simulink model "c00016M_harness"  (R2018a)
settings: Solver=FixedStepAuto  StartTime=0.0  StopTime=300  FixedStep=0.1  RelTol=1e-3
undefined symbols (not defined in the file): A1, hmax, PriorityTank, R1, R2, sigbuilder_block
(part 4 of 24)

== system c00016M_harness/M092 ==
  note: VALUES
      | ---------------------------------
      | ControlType = 1 | 2 | 3
      | FillTank = 0 | 1
      | EmptyTank = 0 | 1
      | ManualReference between 0 and 1
      | Tempreature between 0 and 100
      | EmergencyButton = 0 | 1
      | LiquidLevel between 0 and 1 (hmax)
  note: Inputs For Tank2
  note: NAMES
      | --------------------------------------------
      | CT1 = ControlType Tank 1
      | F1 = Fill Tank 1
      | E1 = Empty Tank 1
      | MR1 = Manual Reference Tank1
      | T1 = Temperature Tank 1
      | EB1 = Emergency Button Tank 1
      | LL1 = Liquid Level 1
  note: Inputs For Tank3
  note: Inputs For Tank1
  CT2 : Inport
  T2 : Inport  Port=2
  EB2 : Inport  Port=3
  CT3 : Inport  Port=4
  F3 : Inport  Port=5
  E3 : Inport  Port=6
  T3 : Inport  Port=7
  EB3 : Inport  Port=8
  Tank2 : Subsystem
  Tank3 : Subsystem
  LL2 : Outport
  LL3 : Outport  Port=2
  wires:
  Tank2/1(LL2) -> LL2/1, Tank3/6(LL2)
  Tank3/1(LL3) -> LL3/1, Tank2/4(LL3)
  EB2/1 -> Tank2/3(EB2)
  CT2/1 -> Tank2/1(CT2)
  E3/1 -> Tank3/3(E3)
  T2/1 -> Tank2/2(T2)
  CT3/1 -> Tank3/1(CT3)
  F3/1 -> Tank3/2(F3)
  EB3/1 -> Tank3/5(EB3)
  T3/1 -> Tank3/4(T3)

== system c00016M_harness/M093 ==
  note: VALUES
      | ---------------------------------
      | ControlType = 1 | 2 | 3
      | FillTank = 0 | 1
      | EmptyTank = 0 | 1
      | ManualReference between 0 and 1
      | Tempreature between 0 and 100
      | EmergencyButton = 0 | 1
      | LiquidLevel between 0 and 1 (hmax)
  note: Inputs For Tank2
  note: NAMES
      | --------------------------------------------
      | CT1 = ControlType Tank 1
      | F1 = Fill Tank 1
      | E1 = Empty Tank 1
      | MR1 = Manual Reference Tank1
      | T1 = Temperature Tank 1
      | EB1 = Emergency Button Tank 1
      | LL1 = Liquid Level 1
  note: Inputs For Tank3
  note: Inputs For Tank1
  CT2 : Inport
  T2 : Inport  Port=2
  EB2 : Inport  Port=3
  CT3 : Inport  Port=4
  F3 : Inport  Port=5
  E3 : Inport  Port=6
  T3 : Inport  Port=7
  EB3 : Inport  Port=8
  Tank2 : Subsystem
  Tank3 : Subsystem
  LL2 : Outport
  LL3 : Outport  Port=2
  wires:
  Tank2/1(LL2) -> LL2/1, Tank3/6(LL2)
  Tank3/1(LL3) -> LL3/1, Tank2/4(LL3)
  EB2/1 -> Tank2/3(EB2)
  CT2/1 -> Tank2/1(CT2)
  E3/1 -> Tank3/3(E3)
  T2/1 -> Tank2/2(T2)
  CT3/1 -> Tank3/1(CT3)
  F3/1 -> Tank3/2(F3)
  EB3/1 -> Tank3/5(EB3)
  T3/1 -> Tank3/4(T3)

== system c00016M_harness/M094 ==
  note: VALUES
      | ---------------------------------
      | ControlType = 1 | 2 | 3
      | FillTank = 0 | 1
      | EmptyTank = 0 | 1
      | ManualReference between 0 and 1
      | Tempreature between 0 and 100
      | EmergencyButton = 0 | 1
      | LiquidLevel between 0 and 1 (hmax)
  note: Inputs For Tank2
  note: NAMES
      | --------------------------------------------
      | CT1 = ControlType Tank 1
      | F1 = Fill Tank 1
      | E1 = Empty Tank 1
      | MR1 = Manual Reference Tank1
      | T1 = Temperature Tank 1
      | EB1 = Emergency Button Tank 1
      | LL1 = Liquid Level 1
  note: Inputs For Tank3
  note: Inputs For Tank1
  CT2 : Inport
  T2 : Inport  Port=2
  EB2 : Inport  Port=3
  CT3 : Inport  Port=4
  F3 : Inport  Port=5
  E3 : Inport  Port=6
  T3 : Inport  Port=7
  EB3 : Inport  Port=8
  Tank2 : Subsystem
  Tank3 : Subsystem
  LL2 : Outport
  LL3 : Outport  Port=2
  wires:
  Tank2/1(LL2) -> LL2/1, Tank3/6(LL2)
  Tank3/1(LL3) -> LL3/1, Tank2/4(LL3)
  EB2/1 -> Tank2/3(EB2)
  CT2/1 -> Tank2/1(CT2)
  E3/1 -> Tank3/3(E3)
  T2/1 -> Tank2/2(T2)
  CT3/1 -> Tank3/1(CT3)
  F3/1 -> Tank3/2(F3)
  EB3/1 -> Tank3/5(EB3)
  T3/1 -> Tank3/4(T3)

== system c00016M_harness/M095 ==
  note: VALUES
      | ---------------------------------
      | ControlType = 1 | 2 | 3
      | FillTank = 0 | 1
      | EmptyTank = 0 | 1
      | ManualReference between 0 and 1
      | Tempreature between 0 and 100
      | EmergencyButton = 0 | 1
      | LiquidLevel between 0 and 1 (hmax)
  note: Inputs For Tank2
  note: NAMES
      | --------------------------------------------
      | CT1 = ControlType Tank 1
      | F1 = Fill Tank 1
      | E1 = Empty Tank 1
      | MR1 = Manual Reference Tank1
      | T1 = Temperature Tank 1
      | EB1 = Emergency Button Tank 1
      | LL1 = Liquid Level 1
  note: Inputs For Tank3
  note: Inputs For Tank1
  CT2 : Inport
  T2 : Inport  Port=2
  EB2 : Inport  Port=3
  CT3 : Inport  Port=4
  F3 : Inport  Port=5
  E3 : Inport  Port=6
  T3 : Inport  Port=7
  EB3 : Inport  Port=8
  Tank2 : Subsystem
  Tank3 : Subsystem
  LL2 : Outport
  LL3 : Outport  Port=2
  wires:
  Tank2/1(LL2) -> LL2/1, Tank3/6(LL2)
  Tank3/1(LL3) -> LL3/1, Tank2/4(LL3)
  EB2/1 -> Tank2/3(EB2)
  CT2/1 -> Tank2/1(CT2)
  E3/1 -> Tank3/3(E3)
  T2/1 -> Tank2/2(T2)
  CT3/1 -> Tank3/1(CT3)
  F3/1 -> Tank3/2(F3)
  EB3/1 -> Tank3/5(EB3)
  T3/1 -> Tank3/4(T3)

== system c00016M_harness/M096 ==
  note: VALUES
      | ---------------------------------
      | ControlType = 1 | 2 | 3
      | FillTank = 0 | 1
      | EmptyTank = 0 | 1
      | ManualReference between 0 and 1
      | Tempreature between 0 and 100
      | EmergencyButton = 0 | 1
      | LiquidLevel between 0 and 1 (hmax)
  note: Inputs For Tank2
  note: NAMES
      | --------------------------------------------
      | CT1 = ControlType Tank 1
      | F1 = Fill Tank 1
      | E1 = Empty Tank 1
      | MR1 = Manual Reference Tank1
      | T1 = Temperature Tank 1
      | EB1 = Emergency Button Tank 1
      | LL1 = Liquid Level 1
  note: Inputs For Tank3
  note: Inputs For Tank1
  CT2 : Inport
  T2 : Inport  Port=2
  EB2 : Inport  Port=3
  CT3 : Inport  Port=4
  F3 : Inport  Port=5
  E3 : Inport  Port=6
  T3 : Inport  Port=7
  EB3 : Inport  Port=8
  Tank2 : Subsystem
  Tank3 : Subsystem
  LL2 : Outport
  LL3 : Outport  Port=2
  wires:
  Tank2/1(LL2) -> LL2/1, Tank3/6(LL2)
  Tank3/1(LL3) -> LL3/1, Tank2/4(LL3)
  EB2/1 -> Tank2/3(EB2)
  CT2/1 -> Tank2/1(CT2)
  E3/1 -> Tank3/3(E3)
  T2/1 -> Tank2/2(T2)
  CT3/1 -> Tank3/1(CT3)
  F3/1 -> Tank3/2(F3)
  EB3/1 -> Tank3/5(EB3)
  T3/1 -> Tank3/4(T3)

== system c00016M_harness/M097 ==
  note: VALUES
      | ---------------------------------
      | ControlType = 1 | 2 | 3
      | FillTank = 0 | 1
      | EmptyTank = 0 | 1
      | ManualReference between 0 and 1
      | Tempreature between 0 and 100
      | EmergencyButton = 0 | 1
      | LiquidLevel between 0 and 1 (hmax)
  note: Inputs For Tank2
  note: NAMES
      | --------------------------------------------
      | CT1 = ControlType Tank 1
      | F1 = Fill Tank 1
      | E1 = Empty Tank 1
      | MR1 = Manual Reference Tank1
      | T1 = Temperature Tank 1
      | EB1 = Emergency Button Tank 1
      | LL1 = Liquid Level 1
  note: Inputs For Tank3
  note: Inputs For Tank1
  CT2 : Inport
  T2 : Inport  Port=2
  EB2 : Inport  Port=3
  CT3 : Inport  Port=4
  F3 : Inport  Port=5
  E3 : Inport  Port=6
  T3 : Inport  Port=7
  EB3 : Inport  Port=8
  Tank2 : Subsystem
  Tank3 : Subsystem
  LL2 : Outport
  LL3 : Outport  Port=2
  wires:
  Tank2/1(LL2) -> LL2/1, Tank3/6(LL2)
  Tank3/1(LL3) -> LL3/1, Tank2/4(LL3)
  EB2/1 -> Tank2/3(EB2)
  CT2/1 -> Tank2/1(CT2)
  E3/1 -> Tank3/3(E3)
  T2/1 -> Tank2/2(T2)
  CT3/1 -> Tank3/1(CT3)
  F3/1 -> Tank3/2(F3)
  EB3/1 -> Tank3/5(EB3)
  T3/1 -> Tank3/4(T3)

== system c00016M_harness/M098 ==
  note: VALUES
      | ---------------------------------
      | ControlType = 1 | 2 | 3
      | FillTank = 0 | 1
      | EmptyTank = 0 | 1
      | ManualReference between 0 and 1
      | Tempreature between 0 and 100
      | EmergencyButton = 0 | 1
      | LiquidLevel between 0 and 1 (hmax)
  note: Inputs For Tank2
  note: NAMES
      | --------------------------------------------
      | CT1 = ControlType Tank 1
      | F1 = Fill Tank 1
      | E1 = Empty Tank 1
      | MR1 = Manual Reference Tank1
      | T1 = Temperature Tank 1
      | EB1 = Emergency Button Tank 1
      | LL1 = Liquid Level 1
  note: Inputs For Tank3
  note: Inputs For Tank1
  CT2 : Inport
  T2 : Inport  Port=2
  EB2 : Inport  Port=3
  CT3 : Inport  Port=4
  F3 : Inport  Port=5
  E3 : Inport  Port=6
  T3 : Inport  Port=7
  EB3 : Inport  Port=8
  Tank2 : Subsystem
  Tank3 : Subsystem
  LL2 : Outport
  LL3 : Outport  Port=2
  wires:
  Tank2/1(LL2) -> LL2/1, Tank3/6(LL2)
  Tank3/1(LL3) -> LL3/1, Tank2/4(LL3)
  EB2/1 -> Tank2/3(EB2)
  CT2/1 -> Tank2/1(CT2)
  E3/1 -> Tank3/3(E3)
  T2/1 -> Tank2/2(T2)
  CT3/1 -> Tank3/1(CT3)
  F3/1 -> Tank3/2(F3)
  EB3/1 -> Tank3/5(EB3)
  T3/1 -> Tank3/4(T3)

== system c00016M_harness/M099 ==
  note: VALUES
      | ---------------------------------
      | ControlType = 1 | 2 | 3
      | FillTank = 0 | 1
      | EmptyTank = 0 | 1
      | ManualReference between 0 and 1
      | Tempreature between 0 and 100
      | EmergencyButton = 0 | 1
      | LiquidLevel between 0 and 1 (hmax)
  note: Inputs For Tank2
  note: NAMES
      | --------------------------------------------
      | CT1 = ControlType Tank 1
      | F1 = Fill Tank 1
      | E1 = Empty Tank 1
      | MR1 = Manual Reference Tank1
      | T1 = Temperature Tank 1
      | EB1 = Emergency Button Tank 1
      | LL1 = Liquid Level 1
  note: Inputs For Tank3
  note: Inputs For Tank1
  CT2 : Inport
  T2 : Inport  Port=2
  EB2 : Inport  Port=3
  CT3 : Inport  Port=4
  F3 : Inport  Port=5
  E3 : Inport  Port=6
  T3 : Inport  Port=7
  EB3 : Inport  Port=8
  Tank2 : Subsystem
  Tank3 : Subsystem
  LL2 : Outport
  LL3 : Outport  Port=2
  wires:
  Tank2/1(LL2) -> LL2/1, Tank3/6(LL2)
  Tank3/1(LL3) -> LL3/1, Tank2/4(LL3)
  EB2/1 -> Tank2/3(EB2)
  CT2/1 -> Tank2/1(CT2)
  E3/1 -> Tank3/3(E3)
  T2/1 -> Tank2/2(T2)
  CT3/1 -> Tank3/1(CT3)
  F3/1 -> Tank3/2(F3)
  EB3/1 -> Tank3/5(EB3)
  T3/1 -> Tank3/4(T3)

== system c00016M_harness/M100 ==
  note: VALUES
      | ---------------------------------
      | ControlType = 1 | 2 | 3
      | FillTank = 0 | 1
      | EmptyTank = 0 | 1
      | ManualReference between 0 and 1
      | Tempreature between 0 and 100
      | EmergencyButton = 0 | 1
      | LiquidLevel between 0 and 1 (hmax)
  note: Inputs For Tank2
  note: NAMES
      | --------------------------------------------
      | CT1 = ControlType Tank 1
      | F1 = Fill Tank 1
      | E1 = Empty Tank 1
      | MR1 = Manual Reference Tank1
      | T1 = Temperature Tank 1
      | EB1 = Emergency Button Tank 1
      | LL1 = Liquid Level 1
  note: Inputs For Tank3
  note: Inputs For Tank1
  CT2 : Inport
  T2 : Inport  Port=2
  EB2 : Inport  Port=3
  CT3 : Inport  Port=4
  F3 : Inport  Port=5
  E3 : Inport  Port=6
  T3 : Inport  Port=7
  EB3 : Inport  Port=8
  Tank2 : Subsystem
  Tank3 : Subsystem
  LL2 : Outport
  LL3 : Outport  Port=2
  wires:
  Tank2/1(LL2) -> LL2/1, Tank3/6(LL2)
  Tank3/1(LL3) -> LL3/1, Tank2/4(LL3)
  EB2/1 -> Tank2/3(EB2)
  CT2/1 -> Tank2/1(CT2)
  E3/1 -> Tank3/3(E3)
  T2/1 -> Tank2/2(T2)
  CT3/1 -> Tank3/1(CT3)
  F3/1 -> Tank3/2(F3)
  EB3/1 -> Tank3/5(EB3)
  T3/1 -> Tank3/4(T3)

== system c00016M_harness/M101 ==
  note: VALUES
      | ---------------------------------
      | ControlType = 1 | 2 | 3
      | FillTank = 0 | 1
      | EmptyTank = 0 | 1
      | ManualReference between 0 and 1
      | Tempreature between 0 and 100
      | EmergencyButton = 0 | 1
      | LiquidLevel between 0 and 1 (hmax)
  note: Inputs For Tank2
  note: NAMES
      | --------------------------------------------
      | CT1 = ControlType Tank 1
      | F1 = Fill Tank 1
      | E1 = Empty Tank 1
      | MR1 = Manual Reference Tank1
      | T1 = Temperature Tank 1
      | EB1 = Emergency Button Tank 1
      | LL1 = Liquid Level 1
  note: Inputs For Tank3
  note: Inputs For Tank1
  CT2 : Inport
  T2 : Inport  Port=2
  EB2 : Inport  Port=3
  CT3 : Inport  Port=4
  F3 : Inport  Port=5
  E3 : Inport  Port=6
  T3 : Inport  Port=7
  EB3 : Inport  Port=8
  Tank2 : Subsystem
  Tank3 : Subsystem
  LL2 : Outport
  LL3 : Outport  Port=2
  wires:
  Tank2/1(LL2) -> LL2/1, Tank3/6(LL2)
  Tank3/1(LL3) -> LL3/1, Tank2/4(LL3)
  EB2/1 -> Tank2/3(EB2)
  CT2/1 -> Tank2/1(CT2)
  E3/1 -> Tank3/3(E3)
  T2/1 -> Tank2/2(T2)
  CT3/1 -> Tank3/1(CT3)
  F3/1 -> Tank3/2(F3)
  EB3/1 -> Tank3/5(EB3)
  T3/1 -> Tank3/4(T3)

== system c00016M_harness/M102 ==
  note: VALUES
      | ---------------------------------
      | ControlType = 1 | 2 | 3
      | FillTank = 0 | 1
      | EmptyTank = 0 | 1
      | ManualReference between 0 and 1
      | Tempreature between 0 and 100
      | EmergencyButton = 0 | 1
      | LiquidLevel between 0 and 1 (hmax)
  note: Inputs For Tank2
  note: NAMES
      | --------------------------------------------
      | CT1 = ControlType Tank 1
      | F1 = Fill Tank 1
      | E1 = Empty Tank 1
      | MR1 = Manual Reference Tank1
      | T1 = Temperature Tank 1
      | EB1 = Emergency Button Tank 1
      | LL1 = Liquid Level 1
  note: Inputs For Tank3
  note: Inputs For Tank1
  CT2 : Inport
  T2 : Inport  Port=2
  EB2 : Inport  Port=3
  CT3 : Inport  Port=4
  F3 : Inport  Port=5
  E3 : Inport  Port=6
  T3 : Inport  Port=7
  EB3 : Inport  Port=8
  Tank2 : Subsystem
  Tank3 : Subsystem
  LL2 : Outport
  LL3 : Outport  Port=2
  wires:
  Tank2/1(LL2) -> LL2/1, Tank3/6(LL2)
  Tank3/1(LL3) -> LL3/1, Tank2/4(LL3)
  EB2/1 -> Tank2/3(EB2)
  CT2/1 -> Tank2/1(CT2)
  E3/1 -> Tank3/3(E3)
  T2/1 -> Tank2/2(T2)
  CT3/1 -> Tank3/1(CT3)
  F3/1 -> Tank3/2(F3)
  EB3/1 -> Tank3/5(EB3)
  T3/1 -> Tank3/4(T3)

== system c00016M_harness/M103 ==
  note: VALUES
      | ---------------------------------
      | ControlType = 1 | 2 | 3
      | FillTank = 0 | 1
      | EmptyTank = 0 | 1
      | ManualReference between 0 and 1
      | Tempreature between 0 and 100
      | EmergencyButton = 0 | 1
      | LiquidLevel between 0 and 1 (hmax)
  note: Inputs For Tank2
  note: NAMES
      | --------------------------------------------
      | CT1 = ControlType Tank 1
      | F1 = Fill Tank 1
      | E1 = Empty Tank 1
      | MR1 = Manual Reference Tank1
      | T1 = Temperature Tank 1
      | EB1 = Emergency Button Tank 1
      | LL1 = Liquid Level 1
  note: Inputs For Tank3
  note: Inputs For Tank1
  CT2 : Inport
  T2 : Inport  Port=2
  EB2 : Inport  Port=3
  CT3 : Inport  Port=4
  F3 : Inport  Port=5
  E3 : Inport  Port=6
  T3 : Inport  Port=7
  EB3 : Inport  Port=8
  Tank2 : Subsystem
  Tank3 : Subsystem
  LL2 : Outport
  LL3 : Outport  Port=2
  wires:
  Tank2/1(LL2) -> LL2/1, Tank3/6(LL2)
  Tank3/1(LL3) -> LL3/1, Tank2/4(LL3)
  EB2/1 -> Tank2/3(EB2)
  CT2/1 -> Tank2/1(CT2)
  E3/1 -> Tank3/3(E3)
  T2/1 -> Tank2/2(T2)
  CT3/1 -> Tank3/1(CT3)
  F3/1 -> Tank3/2(F3)
  EB3/1 -> Tank3/5(EB3)
  T3/1 -> Tank3/4(T3)

== system c00016M_harness/M104 ==
  note: VALUES
      | ---------------------------------
      | ControlType = 1 | 2 | 3
      | FillTank = 0 | 1
      | EmptyTank = 0 | 1
      | ManualReference between 0 and 1
      | Tempreature between 0 and 100
      | EmergencyButton = 0 | 1
      | LiquidLevel between 0 and 1 (hmax)
  note: Inputs For Tank2
  note: NAMES
      | --------------------------------------------
      | CT1 = ControlType Tank 1
      | F1 = Fill Tank 1
      | E1 = Empty Tank 1
      | MR1 = Manual Reference Tank1
      | T1 = Temperature Tank 1
      | EB1 = Emergency Button Tank 1
      | LL1 = Liquid Level 1
  note: Inputs For Tank3
  note: Inputs For Tank1
  CT2 : Inport
  T2 : Inport  Port=2
  EB2 : Inport  Port=3
  CT3 : Inport  Port=4
  F3 : Inport  Port=5
  E3 : Inport  Port=6
  T3 : Inport  Port=7
  EB3 : Inport  Port=8
  Tank2 : Subsystem
  Tank3 : Subsystem
  LL2 : Outport
  LL3 : Outport  Port=2
  wires:
  Tank2/1(LL2) -> LL2/1, Tank3/6(LL2)
  Tank3/1(LL3) -> LL3/1, Tank2/4(LL3)
  EB2/1 -> Tank2/3(EB2)
  CT2/1 -> Tank2/1(CT2)
  E3/1 -> Tank3/3(E3)
  T2/1 -> Tank2/2(T2)
  CT3/1 -> Tank3/1(CT3)
  F3/1 -> Tank3/2(F3)
  EB3/1 -> Tank3/5(EB3)
  T3/1 -> Tank3/4(T3)

== system c00016M_harness/M105 ==
  note: VALUES
      | ---------------------------------
      | ControlType = 1 | 2 | 3
      | FillTank = 0 | 1
      | EmptyTank = 0 | 1
      | ManualReference between 0 and 1
      | Tempreature between 0 and 100
      | EmergencyButton = 0 | 1
      | LiquidLevel between 0 and 1 (hmax)
  note: Inputs For Tank2
  note: NAMES
      | --------------------------------------------
      | CT1 = ControlType Tank 1
      | F1 = Fill Tank 1
      | E1 = Empty Tank 1
      | MR1 = Manual Reference Tank1
      | T1 = Temperature Tank 1
      | EB1 = Emergency Button Tank 1
      | LL1 = Liquid Level 1
  note: Inputs For Tank3
  note: Inputs For Tank1
  CT2 : Inport
  T2 : Inport  Port=2
  EB2 : Inport  Port=3
  CT3 : Inport  Port=4
  F3 : Inport  Port=5
  E3 : Inport  Port=6
  T3 : Inport  Port=7
  EB3 : Inport  Port=8
  Tank2 : Subsystem
  Tank3 : Subsystem
  LL2 : Outport
  LL3 : Outport  Port=2
  wires:
  Tank2/1(LL2) -> LL2/1, Tank3/6(LL2)
  Tank3/1(LL3) -> LL3/1, Tank2/4(LL3)
  EB2/1 -> Tank2/3(EB2)
  CT2/1 -> Tank2/1(CT2)
  E3/1 -> Tank3/3(E3)
  T2/1 -> Tank2/2(T2)
  CT3/1 -> Tank3/1(CT3)
  F3/1 -> Tank3/2(F3)
  EB3/1 -> Tank3/5(EB3)
  T3/1 -> Tank3/4(T3)

== system c00016M_harness/M106 ==
  note: VALUES
      | ---------------------------------
      | ControlType = 1 | 2 | 3
      | FillTank = 0 | 1
      | EmptyTank = 0 | 1
      | ManualReference between 0 and 1
      | Tempreature between 0 and 100
      | EmergencyButton = 0 | 1
      | LiquidLevel between 0 and 1 (hmax)
  note: Inputs For Tank2
  note: NAMES
      | --------------------------------------------
      | CT1 = ControlType Tank 1
      | F1 = Fill Tank 1
      | E1 = Empty Tank 1
      | MR1 = Manual Reference Tank1
      | T1 = Temperature Tank 1
      | EB1 = Emergency Button Tank 1
      | LL1 = Liquid Level 1
  note: Inputs For Tank3
  note: Inputs For Tank1
  CT2 : Inport
  T2 : Inport  Port=2
  EB2 : Inport  Port=3
  CT3 : Inport  Port=4
  F3 : Inport  Port=5
  E3 : Inport  Port=6
  T3 : Inport  Port=7
  EB3 : Inport  Port=8
  Tank2 : Subsystem
  Tank3 : Subsystem
  LL2 : Outport
  LL3 : Outport  Port=2
  wires:
  Tank2/1(LL2) -> LL2/1, Tank3/6(LL2)
  Tank3/1(LL3) -> LL3/1, Tank2/4(LL3)
  EB2/1 -> Tank2/3(EB2)
  CT2/1 -> Tank2/1(CT2)
  E3/1 -> Tank3/3(E3)
  T2/1 -> Tank2/2(T2)
  CT3/1 -> Tank3/1(CT3)
  F3/1 -> Tank3/2(F3)
  EB3/1 -> Tank3/5(EB3)
  T3/1 -> Tank3/4(T3)

== system c00016M_harness/M107 ==
  note: VALUES
      | ---------------------------------
      | ControlType = 1 | 2 | 3
      | FillTank = 0 | 1
      | EmptyTank = 0 | 1
      | ManualReference between 0 and 1
      | Tempreature between 0 and 100
      | EmergencyButton = 0 | 1
      | LiquidLevel between 0 and 1 (hmax)
  note: Inputs For Tank2
  note: NAMES
      | --------------------------------------------
      | CT1 = ControlType Tank 1
      | F1 = Fill Tank 1
      | E1 = Empty Tank 1
      | MR1 = Manual Reference Tank1
      | T1 = Temperature Tank 1
      | EB1 = Emergency Button Tank 1
      | LL1 = Liquid Level 1
  note: Inputs For Tank3
  note: Inputs For Tank1
  CT2 : Inport
  T2 : Inport  Port=2
  EB2 : Inport  Port=3
  CT3 : Inport  Port=4
  F3 : Inport  Port=5
  E3 : Inport  Port=6
  T3 : Inport  Port=7
  EB3 : Inport  Port=8
  Tank2 : Subsystem
  Tank3 : Subsystem
  LL2 : Outport
  LL3 : Outport  Port=2
  wires:
  Tank2/1(LL2) -> LL2/1, Tank3/6(LL2)
  Tank3/1(LL3) -> LL3/1, Tank2/4(LL3)
  EB2/1 -> Tank2/3(EB2)
  CT2/1 -> Tank2/1(CT2)
  E3/1 -> Tank3/3(E3)
  T2/1 -> Tank2/2(T2)
  CT3/1 -> Tank3/1(CT3)
  F3/1 -> Tank3/2(F3)
  EB3/1 -> Tank3/5(EB3)
  T3/1 -> Tank3/4(T3)

== system c00016M_harness/M108 ==
  note: VALUES
      | ---------------------------------
      | ControlType = 1 | 2 | 3
      | FillTank = 0 | 1
      | EmptyTank = 0 | 1
      | ManualReference between 0 and 1
      | Tempreature between 0 and 100
      | EmergencyButton = 0 | 1
      | LiquidLevel between 0 and 1 (hmax)
  note: Inputs For Tank2
  note: NAMES
      | --------------------------------------------
      | CT1 = ControlType Tank 1
      | F1 = Fill Tank 1
      | E1 = Empty Tank 1
      | MR1 = Manual Reference Tank1
      | T1 = Temperature Tank 1
      | EB1 = Emergency Button Tank 1
      | LL1 = Liquid Level 1
  note: Inputs For Tank3
  note: Inputs For Tank1
  CT2 : Inport
  T2 : Inport  Port=2
  EB2 : Inport  Port=3
  CT3 : Inport  Port=4
  F3 : Inport  Port=5
  E3 : Inport  Port=6
  T3 : Inport  Port=7
  EB3 : Inport  Port=8
  Tank2 : Subsystem
  Tank3 : Subsystem
  LL2 : Outport
  LL3 : Outport  Port=2
  wires:
  Tank2/1(LL2) -> LL2/1, Tank3/6(LL2)
  Tank3/1(LL3) -> LL3/1, Tank2/4(LL3)
  EB2/1 -> Tank2/3(EB2)
  CT2/1 -> Tank2/1(CT2)
  E3/1 -> Tank3/3(E3)
  T2/1 -> Tank2/2(T2)
  CT3/1 -> Tank3/1(CT3)
  F3/1 -> Tank3/2(F3)
  EB3/1 -> Tank3/5(EB3)
  T3/1 -> Tank3/4(T3)

== system c00016M_harness/M109 ==
  note: VALUES
      | ---------------------------------
      | ControlType = 1 | 2 | 3
      | FillTank = 0 | 1
      | EmptyTank = 0 | 1
      | ManualReference between 0 and 1
      | Tempreature between 0 and 100
      | EmergencyButton = 0 | 1
      | LiquidLevel between 0 and 1 (hmax)
  note: Inputs For Tank2
  note: NAMES
      | --------------------------------------------
      | CT1 = ControlType Tank 1
      | F1 = Fill Tank 1
      | E1 = Empty Tank 1
      | MR1 = Manual Reference Tank1
      | T1 = Temperature Tank 1
      | EB1 = Emergency Button Tank 1
      | LL1 = Liquid Level 1
  note: Inputs For Tank3
  note: Inputs For Tank1
  CT2 : Inport
  T2 : Inport  Port=2
  EB2 : Inport  Port=3
  CT3 : Inport  Port=4
  F3 : Inport  Port=5
  E3 : Inport  Port=6
  T3 : Inport  Port=7
  EB3 : Inport  Port=8
  Tank2 : Subsystem
  Tank3 : Subsystem
  LL2 : Outport
  LL3 : Outport  Port=2
  wires:
  Tank2/1(LL2) -> LL2/1, Tank3/6(LL2)
  Tank3/1(LL3) -> LL3/1, Tank2/4(LL3)
  EB2/1 -> Tank2/3(EB2)
  CT2/1 -> Tank2/1(CT2)
  E3/1 -> Tank3/3(E3)
  T2/1 -> Tank2/2(T2)
  CT3/1 -> Tank3/1(CT3)
  F3/1 -> Tank3/2(F3)
  EB3/1 -> Tank3/5(EB3)
  T3/1 -> Tank3/4(T3)

== system c00016M_harness/M110 ==
  note: VALUES
      | ---------------------------------
      | ControlType = 1 | 2 | 3
      | FillTank = 0 | 1
      | EmptyTank = 0 | 1
      | ManualReference between 0 and 1
      | Tempreature between 0 and 100
      | EmergencyButton = 0 | 1
      | LiquidLevel between 0 and 1 (hmax)
  note: Inputs For Tank2
  note: NAMES
      | --------------------------------------------
      | CT1 = ControlType Tank 1
      | F1 = Fill Tank 1
      | E1 = Empty Tank 1
      | MR1 = Manual Reference Tank1
      | T1 = Temperature Tank 1
      | EB1 = Emergency Button Tank 1
      | LL1 = Liquid Level 1
  note: Inputs For Tank3
  note: Inputs For Tank1
  CT2 : Inport
  T2 : Inport  Port=2
  EB2 : Inport  Port=3
  CT3 : Inport  Port=4
  F3 : Inport  Port=5
  E3 : Inport  Port=6
  T3 : Inport  Port=7
  EB3 : Inport  Port=8
  Tank2 : Subsystem
  Tank3 : Subsystem
  LL2 : Outport
  LL3 : Outport  Port=2
  wires:
  Tank2/1(LL2) -> LL2/1, Tank3/6(LL2)
  Tank3/1(LL3) -> LL3/1, Tank2/4(LL3)
  EB2/1 -> Tank2/3(EB2)
  CT2/1 -> Tank2/1(CT2)
  E3/1 -> Tank3/3(E3)
  T2/1 -> Tank2/2(T2)
  CT3/1 -> Tank3/1(CT3)
  F3/1 -> Tank3/2(F3)
  EB3/1 -> Tank3/5(EB3)
  T3/1 -> Tank3/4(T3)

== system c00016M_harness/M111 ==
  note: VALUES
      | ---------------------------------
      | ControlType = 1 | 2 | 3
      | FillTank = 0 | 1
      | EmptyTank = 0 | 1
      | ManualReference between 0 and 1
      | Tempreature between 0 and 100
      | EmergencyButton = 0 | 1
      | LiquidLevel between 0 and 1 (hmax)
  note: Inputs For Tank2
  note: NAMES
      | --------------------------------------------
      | CT1 = ControlType Tank 1
      | F1 = Fill Tank 1
      | E1 = Empty Tank 1
      | MR1 = Manual Reference Tank1
      | T1 = Temperature Tank 1
      | EB1 = Emergency Button Tank 1
      | LL1 = Liquid Level 1
  note: Inputs For Tank3
  note: Inputs For Tank1
  CT2 : Inport
  T2 : Inport  Port=2
  EB2 : Inport  Port=3
  CT3 : Inport  Port=4
  F3 : Inport  Port=5
  E3 : Inport  Port=6
  T3 : Inport  Port=7
  EB3 : Inport  Port=8
  Tank2 : Subsystem
  Tank3 : Subsystem
  LL2 : Outport
  LL3 : Outport  Port=2
  wires:
  Tank2/1(LL2) -> LL2/1, Tank3/6(LL2)
  Tank3/1(LL3) -> LL3/1, Tank2/4(LL3)
  EB2/1 -> Tank2/3(EB2)
  CT2/1 -> Tank2/1(CT2)
  E3/1 -> Tank3/3(E3)
  T2/1 -> Tank2/2(T2)
  CT3/1 -> Tank3/1(CT3)
  F3/1 -> Tank3/2(F3)
  EB3/1 -> Tank3/5(EB3)
  T3/1 -> Tank3/4(T3)

== system c00016M_harness/M112 ==
  note: VALUES
      | ---------------------------------
      | ControlType = 1 | 2 | 3
      | FillTank = 0 | 1
      | EmptyTank = 0 | 1
      | ManualReference between 0 and 1
      | Tempreature between 0 and 100
      | EmergencyButton = 0 | 1
      | LiquidLevel between 0 and 1 (hmax)
  note: Inputs For Tank2
  note: NAMES
      | --------------------------------------------
      | CT1 = ControlType Tank 1
      | F1 = Fill Tank 1
      | E1 = Empty Tank 1
      | MR1 = Manual Reference Tank1
      | T1 = Temperature Tank 1
      | EB1 = Emergency Button Tank 1
      | LL1 = Liquid Level 1
  note: Inputs For Tank3
  note: Inputs For Tank1
  CT2 : Inport
  T2 : Inport  Port=2
  EB2 : Inport  Port=3
  CT3 : Inport  Port=4
  F3 : Inport  Port=5
  E3 : Inport  Port=6
  T3 : Inport  Port=7
  EB3 : Inport  Port=8
  Tank2 : Subsystem
  Tank3 : Subsystem
  LL2 : Outport
  LL3 : Outport  Port=2
  wires:
  Tank2/1(LL2) -> LL2/1, Tank3/6(LL2)
  Tank3/1(LL3) -> LL3/1, Tank2/4(LL3)
  EB2/1 -> Tank2/3(EB2)
  CT2/1 -> Tank2/1(CT2)
  E3/1 -> Tank3/3(E3)
  T2/1 -> Tank2/2(T2)
  CT3/1 -> Tank3/1(CT3)
  F3/1 -> Tank3/2(F3)
  EB3/1 -> Tank3/5(EB3)
  T3/1 -> Tank3/4(T3)

== system c00016M_harness/M113 ==
  note: VALUES
      | ---------------------------------
      | ControlType = 1 | 2 | 3
      | FillTank = 0 | 1
      | EmptyTank = 0 | 1
      | ManualReference between 0 and 1
      | Tempreature between 0 and 100
      | EmergencyButton = 0 | 1
      | LiquidLevel between 0 and 1 (hmax)
  note: Inputs For Tank2
  note: NAMES
      | --------------------------------------------
      | CT1 = ControlType Tank 1
      | F1 = Fill Tank 1
      | E1 = Empty Tank 1
      | MR1 = Manual Reference Tank1
      | T1 = Temperature Tank 1
      | EB1 = Emergency Button Tank 1
      | LL1 = Liquid Level 1
  note: Inputs For Tank3
  note: Inputs For Tank1
  CT2 : Inport
  T2 : Inport  Port=2
  EB2 : Inport  Port=3
  CT3 : Inport  Port=4
  F3 : Inport  Port=5
  E3 : Inport  Port=6
  T3 : Inport  Port=7
  EB3 : Inport  Port=8
  Tank2 : Subsystem
  Tank3 : Subsystem
  LL2 : Outport
  LL3 : Outport  Port=2
  wires:
  Tank2/1(LL2) -> LL2/1, Tank3/6(LL2)
  Tank3/1(LL3) -> LL3/1, Tank2/4(LL3)
  EB2/1 -> Tank2/3(EB2)
  CT2/1 -> Tank2/1(CT2)
  E3/1 -> Tank3/3(E3)
  T2/1 -> Tank2/2(T2)
  CT3/1 -> Tank3/1(CT3)
  F3/1 -> Tank3/2(F3)
  EB3/1 -> Tank3/5(EB3)
  T3/1 -> Tank3/4(T3)

== system c00016M_harness/M114 ==
  note: VALUES
      | ---------------------------------
      | ControlType = 1 | 2 | 3
      | FillTank = 0 | 1
      | EmptyTank = 0 | 1
      | ManualReference between 0 and 1
      | Tempreature between 0 and 100
      | EmergencyButton = 0 | 1
      | LiquidLevel between 0 and 1 (hmax)
  note: Inputs For Tank2
  note: NAMES
      | --------------------------------------------
      | CT1 = ControlType Tank 1
      | F1 = Fill Tank 1
      | E1 = Empty Tank 1
      | MR1 = Manual Reference Tank1
      | T1 = Temperature Tank 1
      | EB1 = Emergency Button Tank 1
      | LL1 = Liquid Level 1
  note: Inputs For Tank3
  note: Inputs For Tank1
  CT2 : Inport
  T2 : Inport  Port=2
  EB2 : Inport  Port=3
  CT3 : Inport  Port=4
  F3 : Inport  Port=5
  E3 : Inport  Port=6
  T3 : Inport  Port=7
  EB3 : Inport  Port=8
  Tank2 : Subsystem
  Tank3 : Subsystem
  LL2 : Outport
  LL3 : Outport  Port=2
  wires:
  Tank2/1(LL2) -> LL2/1, Tank3/6(LL2)
  Tank3/1(LL3) -> LL3/1, Tank2/4(LL3)
  EB2/1 -> Tank2/3(EB2)
  CT2/1 -> Tank2/1(CT2)
  E3/1 -> Tank3/3(E3)
  T2/1 -> Tank2/2(T2)
  CT3/1 -> Tank3/1(CT3)
  F3/1 -> Tank3/2(F3)
  EB3/1 -> Tank3/5(EB3)
  T3/1 -> Tank3/4(T3)

== system c00016M_harness/M115 ==
  note: VALUES
      | ---------------------------------
      | ControlType = 1 | 2 | 3
      | FillTank = 0 | 1
      | EmptyTank = 0 | 1
      | ManualReference between 0 and 1
      | Tempreature between 0 and 100
      | EmergencyButton = 0 | 1
      | LiquidLevel between 0 and 1 (hmax)
  note: Inputs For Tank2
  note: NAMES
      | --------------------------------------------
      | CT1 = ControlType Tank 1
      | F1 = Fill Tank 1
      | E1 = Empty Tank 1
      | MR1 = Manual Reference Tank1
      | T1 = Temperature Tank 1
      | EB1 = Emergency Button Tank 1
      | LL1 = Liquid Level 1
  note: Inputs For Tank3
  note: Inputs For Tank1
  CT2 : Inport
  T2 : Inport  Port=2
  EB2 : Inport  Port=3
  CT3 : Inport  Port=4
  F3 : Inport  Port=5
  E3 : Inport  Port=6
  T3 : Inport  Port=7
  EB3 : Inport  Port=8
  Tank2 : Subsystem
  Tank3 : Subsystem
  LL2 : Outport
  LL3 : Outport  Port=2
  wires:
  Tank2/1(LL2) -> LL2/1, Tank3/6(LL2)
  Tank3/1(LL3) -> LL3/1, Tank2/4(LL3)
  EB2/1 -> Tank2/3(EB2)
  CT2/1 -> Tank2/1(CT2)
  E3/1 -> Tank3/3(E3)
  T2/1 -> Tank2/2(T2)
  CT3/1 -> Tank3/1(CT3)
  F3/1 -> Tank3/2(F3)
  EB3/1 -> Tank3/5(EB3)
  T3/1 -> Tank3/4(T3)

== system c00016M_harness/M116 ==
  note: VALUES
      | ---------------------------------
      | ControlType = 1 | 2 | 3
      | FillTank = 0 | 1
      | EmptyTank = 0 | 1
      | ManualReference between 0 and 1
      | Tempreature between 0 and 100
      | EmergencyButton = 0 | 1
      | LiquidLevel between 0 and 1 (hmax)
  note: Inputs For Tank2
  note: NAMES
      | --------------------------------------------
      | CT1 = ControlType Tank 1
      | F1 = Fill Tank 1
      | E1 = Empty Tank 1
      | MR1 = Manual Reference Tank1
      | T1 = Temperature Tank 1
      | EB1 = Emergency Button Tank 1
      | LL1 = Liquid Level 1
  note: Inputs For Tank3
  note: Inputs For Tank1
  CT2 : Inport
  T2 : Inport  Port=2
  EB2 : Inport  Port=3
  CT3 : Inport  Port=4
  F3 : Inport  Port=5
  E3 : Inport  Port=6
  T3 : Inport  Port=7
  EB3 : Inport  Port=8
  Tank2 : Subsystem
  Tank3 : Subsystem
  LL2 : Outport
  LL3 : Outport  Port=2
  wires:
  Tank2/1(LL2) -> LL2/1, Tank3/6(LL2)
  Tank3/1(LL3) -> LL3/1, Tank2/4(LL3)
  EB2/1 -> Tank2/3(EB2)
  CT2/1 -> Tank2/1(CT2)
  E3/1 -> Tank3/3(E3)
  T2/1 -> Tank2/2(T2)
  CT3/1 -> Tank3/1(CT3)
  F3/1 -> Tank3/2(F3)
  EB3/1 -> Tank3/5(EB3)
  T3/1 -> Tank3/4(T3)

== system c00016M_harness/M117 ==
  note: VALUES
      | ---------------------------------
      | ControlType = 1 | 2 | 3
      | FillTank = 0 | 1
      | EmptyTank = 0 | 1
      | ManualReference between 0 and 1
      | Tempreature between 0 and 100
      | EmergencyButton = 0 | 1
      | LiquidLevel between 0 and 1 (hmax)
  note: Inputs For Tank2
  note: NAMES
      | --------------------------------------------
      | CT1 = ControlType Tank 1
      | F1 = Fill Tank 1
      | E1 = Empty Tank 1
      | MR1 = Manual Reference Tank1
      | T1 = Temperature Tank 1
      | EB1 = Emergency Button Tank 1
      | LL1 = Liquid Level 1
  note: Inputs For Tank3
  note: Inputs For Tank1
  CT2 : Inport
  T2 : Inport  Port=2
  EB2 : Inport  Port=3
  CT3 : Inport  Port=4
  F3 : Inport  Port=5
  E3 : Inport  Port=6
  T3 : Inport  Port=7
  EB3 : Inport  Port=8
  Tank2 : Subsystem
  Tank3 : Subsystem
  LL2 : Outport
  LL3 : Outport  Port=2
  wires:
  Tank2/1(LL2) -> LL2/1, Tank3/6(LL2)
  Tank3/1(LL3) -> LL3/1, Tank2/4(LL3)
  EB2/1 -> Tank2/3(EB2)
  CT2/1 -> Tank2/1(CT2)
  E3/1 -> Tank3/3(E3)
  T2/1 -> Tank2/2(T2)
  CT3/1 -> Tank3/1(CT3)
  F3/1 -> Tank3/2(F3)
  EB3/1 -> Tank3/5(EB3)
  T3/1 -> Tank3/4(T3)

== system c00016M_harness/M140 ==
  note: VALUES
      | ---------------------------------
      | ControlType = 1 | 2 | 3
      | FillTank = 0 | 1
      | EmptyTank = 0 | 1
      | ManualReference between 0 and 1
      | Tempreature between 0 and 100
      | EmergencyButton = 0 | 1
      | LiquidLevel between 0 and 1 (hmax)
  note: Inputs For Tank2
  note: NAMES
      | --------------------------------------------
      | CT1 = ControlType Tank 1
      | F1 = Fill Tank 1
      | E1 = Empty Tank 1
      | MR1 = Manual Reference Tank1
      | T1 = Temperature Tank 1
      | EB1 = Emergency Button Tank 1
      | LL1 = Liquid Level 1
  note: Inputs For Tank3
  note: Inputs For Tank1
  CT2 : Inport
  T2 : Inport  Port=2
  EB2 : Inport  Port=3
  CT3 : Inport  Port=4
  F3 : Inport  Port=5
  E3 : Inport  Port=6
  T3 : Inport  Port=7
  EB3 : Inport  Port=8
  Tank2 : Subsystem
  Tank3 : Subsystem
  LL2 : Outport
  LL3 : Outport  Port=2
  wires:
  Tank2/1(LL2) -> LL2/1, Tank3/6(LL2)
  Tank3/1(LL3) -> LL3/1, Tank2/4(LL3)
  EB2/1 -> Tank2/3(EB2)
  CT2/1 -> Tank2/1(CT2)
  E3/1 -> Tank3/3(E3)
  T2/1 -> Tank2/2(T2)
  CT3/1 -> Tank3/1(CT3)
  F3/1 -> Tank3/2(F3)
  EB3/1 -> Tank3/5(EB3)
  T3/1 -> Tank3/4(T3)

== system c00016M_harness/M141 ==
  note: VALUES
      | ---------------------------------
      | ControlType = 1 | 2 | 3
      | FillTank = 0 | 1
      | EmptyTank = 0 | 1
      | ManualReference between 0 and 1
      | Tempreature between 0 and 100
      | EmergencyButton = 0 | 1
      | LiquidLevel between 0 and 1 (hmax)
  note: Inputs For Tank2
  note: NAMES
      | --------------------------------------------
      | CT1 = ControlType Tank 1
      | F1 = Fill Tank 1
      | E1 = Empty Tank 1
      | MR1 = Manual Reference Tank1
      | T1 = Temperature Tank 1
      | EB1 = Emergency Button Tank 1
      | LL1 = Liquid Level 1
  note: Inputs For Tank3
  note: Inputs For Tank1
  CT2 : Inport
  T2 : Inport  Port=2
  EB2 : Inport  Port=3
  CT3 : Inport  Port=4
  F3 : Inport  Port=5
  E3 : Inport  Port=6
  T3 : Inport  Port=7
  EB3 : Inport  Port=8
  Tank2 : Subsystem
  Tank3 : Subsystem
  LL2 : Outport
  LL3 : Outport  Port=2
  wires:
  Tank2/1(LL2) -> LL2/1, Tank3/6(LL2)
  Tank3/1(LL3) -> LL3/1, Tank2/4(LL3)
  EB2/1 -> Tank2/3(EB2)
  CT2/1 -> Tank2/1(CT2)
  E3/1 -> Tank3/3(E3)
  T2/1 -> Tank2/2(T2)
  CT3/1 -> Tank3/1(CT3)
  F3/1 -> Tank3/2(F3)
  EB3/1 -> Tank3/5(EB3)
  T3/1 -> Tank3/4(T3)

== system c00016M_harness/M142 ==
  note: VALUES
      | ---------------------------------
      | ControlType = 1 | 2 | 3
      | FillTank = 0 | 1
      | EmptyTank = 0 | 1
      | ManualReference between 0 and 1
      | Tempreature between 0 and 100
      | EmergencyButton = 0 | 1
      | LiquidLevel between 0 and 1 (hmax)
  note: Inputs For Tank2
  note: NAMES
      | --------------------------------------------
      | CT1 = ControlType Tank 1
      | F1 = Fill Tank 1
      | E1 = Empty Tank 1
      | MR1 = Manual Reference Tank1
      | T1 = Temperature Tank 1
      | EB1 = Emergency Button Tank 1
      | LL1 = Liquid Level 1
  note: Inputs For Tank3
  note: Inputs For Tank1
  CT2 : Inport
  T2 : Inport  Port=2
  EB2 : Inport  Port=3
  CT3 : Inport  Port=4
  F3 : Inport  Port=5
  E3 : Inport  Port=6
  T3 : Inport  Port=7
  EB3 : Inport  Port=8
  Tank2 : Subsystem
  Tank3 : Subsystem
  LL2 : Outport
  LL3 : Outport  Port=2
  wires:
  Tank2/1(LL2) -> LL2/1, Tank3/6(LL2)
  Tank3/1(LL3) -> LL3/1, Tank2/4(LL3)
  EB2/1 -> Tank2/3(EB2)
  CT2/1 -> Tank2/1(CT2)
  E3/1 -> Tank3/3(E3)
  T2/1 -> Tank2/2(T2)
  CT3/1 -> Tank3/1(CT3)
  F3/1 -> Tank3/2(F3)
  EB3/1 -> Tank3/5(EB3)
  T3/1 -> Tank3/4(T3)

== system c00016M_harness/M143 ==
  note: VALUES
      | ---------------------------------
      | ControlType = 1 | 2 | 3
      | FillTank = 0 | 1
      | EmptyTank = 0 | 1
      | ManualReference between 0 and 1
      | Tempreature between 0 and 100
      | EmergencyButton = 0 | 1
      | LiquidLevel between 0 and 1 (hmax)
  note: Inputs For Tank2
  note: NAMES
      | --------------------------------------------
      | CT1 = ControlType Tank 1
      | F1 = Fill Tank 1
      | E1 = Empty Tank 1
      | MR1 = Manual Reference Tank1
      | T1 = Temperature Tank 1
      | EB1 = Emergency Button Tank 1
      | LL1 = Liquid Level 1
  note: Inputs For Tank3
  note: Inputs For Tank1
  CT2 : Inport
  T2 : Inport  Port=2
  EB2 : Inport  Port=3
  CT3 : Inport  Port=4
  F3 : Inport  Port=5
  E3 : Inport  Port=6
  T3 : Inport  Port=7
  EB3 : Inport  Port=8
  Tank2 : Subsystem
  Tank3 : Subsystem
  LL2 : Outport
  LL3 : Outport  Port=2
  wires:
  Tank2/1(LL2) -> LL2/1, Tank3/6(LL2)
  Tank3/1(LL3) -> LL3/1, Tank2/4(LL3)
  EB2/1 -> Tank2/3(EB2)
  CT2/1 -> Tank2/1(CT2)
  E3/1 -> Tank3/3(E3)
  T2/1 -> Tank2/2(T2)
  CT3/1 -> Tank3/1(CT3)
  F3/1 -> Tank3/2(F3)
  EB3/1 -> Tank3/5(EB3)
  T3/1 -> Tank3/4(T3)

== system c00016M_harness/M144 ==
  note: VALUES
      | ---------------------------------
      | ControlType = 1 | 2 | 3
      | FillTank = 0 | 1
      | EmptyTank = 0 | 1
      | ManualReference between 0 and 1
      | Tempreature between 0 and 100
      | EmergencyButton = 0 | 1
      | LiquidLevel between 0 and 1 (hmax)
  note: Inputs For Tank2
  note: NAMES
      | --------------------------------------------
      | CT1 = ControlType Tank 1
      | F1 = Fill Tank 1
      | E1 = Empty Tank 1
      | MR1 = Manual Reference Tank1
      | T1 = Temperature Tank 1
      | EB1 = Emergency Button Tank 1
      | LL1 = Liquid Level 1
  note: Inputs For Tank3
  note: Inputs For Tank1
  CT2 : Inport
  T2 : Inport  Port=2
  EB2 : Inport  Port=3
  CT3 : Inport  Port=4
  F3 : Inport  Port=5
  E3 : Inport  Port=6
  T3 : Inport  Port=7
  EB3 : Inport  Port=8
  Tank2 : Subsystem
  Tank3 : Subsystem
  LL2 : Outport
  LL3 : Outport  Port=2
  wires:
  Tank2/1(LL2) -> LL2/1, Tank3/6(LL2)
  Tank3/1(LL3) -> LL3/1, Tank2/4(LL3)
  EB2/1 -> Tank2/3(EB2)
  CT2/1 -> Tank2/1(CT2)
  E3/1 -> Tank3/3(E3)
  T2/1 -> Tank2/2(T2)
  CT3/1 -> Tank3/1(CT3)
  F3/1 -> Tank3/2(F3)
  EB3/1 -> Tank3/5(EB3)
  T3/1 -> Tank3/4(T3)

== system c00016M_harness/M145 ==
  note: VALUES
      | ---------------------------------
      | ControlType = 1 | 2 | 3
      | FillTank = 0 | 1
      | EmptyTank = 0 | 1
      | ManualReference between 0 and 1
      | Tempreature between 0 and 100
      | EmergencyButton = 0 | 1
      | LiquidLevel between 0 and 1 (hmax)
  note: Inputs For Tank2
  note: NAMES
      | --------------------------------------------
      | CT1 = ControlType Tank 1
      | F1 = Fill Tank 1
      | E1 = Empty Tank 1
      | MR1 = Manual Reference Tank1
      | T1 = Temperature Tank 1
      | EB1 = Emergency Button Tank 1
      | LL1 = Liquid Level 1
  note: Inputs For Tank3
  note: Inputs For Tank1
  CT2 : Inport
  T2 : Inport  Port=2
  EB2 : Inport  Port=3
  CT3 : Inport  Port=4
  F3 : Inport  Port=5
  E3 : Inport  Port=6
  T3 : Inport  Port=7
  EB3 : Inport  Port=8
  Tank2 : Subsystem
  Tank3 : Subsystem
  LL2 : Outport
  LL3 : Outport  Port=2
  wires:
  Tank2/1(LL2) -> LL2/1, Tank3/6(LL2)
  Tank3/1(LL3) -> LL3/1, Tank2/4(LL3)
  EB2/1 -> Tank2/3(EB2)
  CT2/1 -> Tank2/1(CT2)
  E3/1 -> Tank3/3(E3)
  T2/1 -> Tank2/2(T2)
  CT3/1 -> Tank3/1(CT3)
  F3/1 -> Tank3/2(F3)
  EB3/1 -> Tank3/5(EB3)
  T3/1 -> Tank3/4(T3)

== system c00016M_harness/M146 ==
  note: VALUES
      | ---------------------------------
      | ControlType = 1 | 2 | 3
      | FillTank = 0 | 1
      | EmptyTank = 0 | 1
      | ManualReference between 0 and 1
      | Tempreature between 0 and 100
      | EmergencyButton = 0 | 1
      | LiquidLevel between 0 and 1 (hmax)
  note: Inputs For Tank2
  note: NAMES
      | --------------------------------------------
      | CT1 = ControlType Tank 1
      | F1 = Fill Tank 1
      | E1 = Empty Tank 1
      | MR1 = Manual Reference Tank1
      | T1 = Temperature Tank 1
      | EB1 = Emergency Button Tank 1
      | LL1 = Liquid Level 1
  note: Inputs For Tank3
  note: Inputs For Tank1
  CT2 : Inport
  T2 : Inport  Port=2
  EB2 : Inport  Port=3
  CT3 : Inport  Port=4
  F3 : Inport  Port=5
  E3 : Inport  Port=6
  T3 : Inport  Port=7
  EB3 : Inport  Port=8
  Tank2 : Subsystem
  Tank3 : Subsystem
  LL2 : Outport
  LL3 : Outport  Port=2
  wires:
  Tank2/1(LL2) -> LL2/1, Tank3/6(LL2)
  Tank3/1(LL3) -> LL3/1, Tank2/4(LL3)
  EB2/1 -> Tank2/3(EB2)
  CT2/1 -> Tank2/1(CT2)
  E3/1 -> Tank3/3(E3)
  T2/1 -> Tank2/2(T2)
  CT3/1 -> Tank3/1(CT3)
  F3/1 -> Tank3/2(F3)
  EB3/1 -> Tank3/5(EB3)
  T3/1 -> Tank3/4(T3)

== system c00016M_harness/M147 ==
  note: VALUES
      | ---------------------------------
      | ControlType = 1 | 2 | 3
      | FillTank = 0 | 1
      | EmptyTank = 0 | 1
      | ManualReference between 0 and 1
      | Tempreature between 0 and 100
      | EmergencyButton = 0 | 1
      | LiquidLevel between 0 and 1 (hmax)
  note: Inputs For Tank2
  note: NAMES
      | --------------------------------------------
      | CT1 = ControlType Tank 1
      | F1 = Fill Tank 1
      | E1 = Empty Tank 1
      | MR1 = Manual Reference Tank1
      | T1 = Temperature Tank 1
      | EB1 = Emergency Button Tank 1
      | LL1 = Liquid Level 1
  note: Inputs For Tank3
  note: Inputs For Tank1
  CT2 : Inport
  T2 : Inport  Port=2
  EB2 : Inport  Port=3
  CT3 : Inport  Port=4
  F3 : Inport  Port=5
  E3 : Inport  Port=6
  T3 : Inport  Port=7
  EB3 : Inport  Port=8
  Tank2 : Subsystem
  Tank3 : Subsystem
  LL2 : Outport
  LL3 : Outport  Port=2
  wires:
  Tank2/1(LL2) -> LL2/1, Tank3/6(LL2)
  Tank3/1(LL3) -> LL3/1, Tank2/4(LL3)
  EB2/1 -> Tank2/3(EB2)
  CT2/1 -> Tank2/1(CT2)
  E3/1 -> Tank3/3(E3)
  T2/1 -> Tank2/2(T2)
  CT3/1 -> Tank3/1(CT3)
  F3/1 -> Tank3/2(F3)
  EB3/1 -> Tank3/5(EB3)
  T3/1 -> Tank3/4(T3)

== system c00016M_harness/M148 ==
  note: VALUES
      | ---------------------------------
      | ControlType = 1 | 2 | 3
      | FillTank = 0 | 1
      | EmptyTank = 0 | 1
      | ManualReference between 0 and 1
      | Tempreature between 0 and 100
      | EmergencyButton = 0 | 1
      | LiquidLevel between 0 and 1 (hmax)
  note: Inputs For Tank2
  note: NAMES
      | --------------------------------------------
      | CT1 = ControlType Tank 1
      | F1 = Fill Tank 1
      | E1 = Empty Tank 1
      | MR1 = Manual Reference Tank1
      | T1 = Temperature Tank 1
      | EB1 = Emergency Button Tank 1
      | LL1 = Liquid Level 1
  note: Inputs For Tank3
  note: Inputs For Tank1
  CT2 : Inport
  T2 : Inport  Port=2
  EB2 : Inport  Port=3
  CT3 : Inport  Port=4
  F3 : Inport  Port=5
  E3 : Inport  Port=6
  T3 : Inport  Port=7
  EB3 : Inport  Port=8
  Tank2 : Subsystem
  Tank3 : Subsystem
  LL2 : Outport
  LL3 : Outport  Port=2
  wires:
  Tank2/1(LL2) -> LL2/1, Tank3/6(LL2)
  Tank3/1(LL3) -> LL3/1, Tank2/4(LL3)
  EB2/1 -> Tank2/3(EB2)
  CT2/1 -> Tank2/1(CT2)
  E3/1 -> Tank3/3(E3)
  T2/1 -> Tank2/2(T2)
  CT3/1 -> Tank3/1(CT3)
  F3/1 -> Tank3/2(F3)
  EB3/1 -> Tank3/5(EB3)
  T3/1 -> Tank3/4(T3)

== system c00016M_harness/M149 ==
  note: VALUES
      | ---------------------------------
      | ControlType = 1 | 2 | 3
      | FillTank = 0 | 1
      | EmptyTank = 0 | 1
      | ManualReference between 0 and 1
      | Tempreature between 0 and 100
      | EmergencyButton = 0 | 1
      | LiquidLevel between 0 and 1 (hmax)
  note: Inputs For Tank2
  note: NAMES
      | --------------------------------------------
      | CT1 = ControlType Tank 1
      | F1 = Fill Tank 1
      | E1 = Empty Tank 1
      | MR1 = Manual Reference Tank1
      | T1 = Temperature Tank 1
      | EB1 = Emergency Button Tank 1
      | LL1 = Liquid Level 1
  note: Inputs For Tank3
  note: Inputs For Tank1
  CT2 : Inport
  T2 : Inport  Port=2
  EB2 : Inport  Port=3
  CT3 : Inport  Port=4
  F3 : Inport  Port=5
  E3 : Inport  Port=6
  T3 : Inport  Port=7
  EB3 : Inport  Port=8
  Tank2 : Subsystem
  Tank3 : Subsystem
  LL2 : Outport
  LL3 : Outport  Port=2
  wires:
  Tank2/1(LL2) -> LL2/1, Tank3/6(LL2)
  Tank3/1(LL3) -> LL3/1, Tank2/4(LL3)
  EB2/1 -> Tank2/3(EB2)
  CT2/1 -> Tank2/1(CT2)
  E3/1 -> Tank3/3(E3)
  T2/1 -> Tank2/2(T2)
  CT3/1 -> Tank3/1(CT3)
  F3/1 -> Tank3/2(F3)
  EB3/1 -> Tank3/5(EB3)
  T3/1 -> Tank3/4(T3)

== system c00016M_harness/M150 ==
  note: VALUES
      | ---------------------------------
      | ControlType = 1 | 2 | 3
      | FillTank = 0 | 1
      | EmptyTank = 0 | 1
      | ManualReference between 0 and 1
      | Tempreature between 0 and 100
      | EmergencyButton = 0 | 1
      | LiquidLevel between 0 and 1 (hmax)
  note: Inputs For Tank2
  note: NAMES
      | --------------------------------------------
      | CT1 = ControlType Tank 1
      | F1 = Fill Tank 1
      | E1 = Empty Tank 1
      | MR1 = Manual Reference Tank1
      | T1 = Temperature Tank 1
      | EB1 = Emergency Button Tank 1
      | LL1 = Liquid Level 1
  note: Inputs For Tank3
  note: Inputs For Tank1
  CT2 : Inport
  T2 : Inport  Port=2
  EB2 : Inport  Port=3
  CT3 : Inport  Port=4
  F3 : Inport  Port=5
  E3 : Inport  Port=6
  T3 : Inport  Port=7
  EB3 : Inport  Port=8
  Tank2 : Subsystem
  Tank3 : Subsystem
  LL2 : Outport
  LL3 : Outport  Port=2
  wires:
  Tank2/1(LL2) -> LL2/1, Tank3/6(LL2)
  Tank3/1(LL3) -> LL3/1, Tank2/4(LL3)
  EB2/1 -> Tank2/3(EB2)
  CT2/1 -> Tank2/1(CT2)
  E3/1 -> Tank3/3(E3)
  T2/1 -> Tank2/2(T2)
  CT3/1 -> Tank3/1(CT3)
  F3/1 -> Tank3/2(F3)
  EB3/1 -> Tank3/5(EB3)
  T3/1 -> Tank3/4(T3)

== system c00016M_harness/M151 ==
  note: VALUES
      | ---------------------------------
      | ControlType = 1 | 2 | 3
      | FillTank = 0 | 1
      | EmptyTank = 0 | 1
      | ManualReference between 0 and 1
      | Tempreature between 0 and 100
      | EmergencyButton = 0 | 1
      | LiquidLevel between 0 and 1 (hmax)
  note: Inputs For Tank2
  note: NAMES
      | --------------------------------------------
      | CT1 = ControlType Tank 1
      | F1 = Fill Tank 1
      | E1 = Empty Tank 1
      | MR1 = Manual Reference Tank1
      | T1 = Temperature Tank 1
      | EB1 = Emergency Button Tank 1
      | LL1 = Liquid Level 1
  note: Inputs For Tank3
  note: Inputs For Tank1
  CT2 : Inport
  T2 : Inport  Port=2
  EB2 : Inport  Port=3
  CT3 : Inport  Port=4
  F3 : Inport  Port=5
  E3 : Inport  Port=6
  T3 : Inport  Port=7
  EB3 : Inport  Port=8
  Tank2 : Subsystem
  Tank3 : Subsystem
  LL2 : Outport
  LL3 : Outport  Port=2
  wires:
  Tank2/1(LL2) -> LL2/1, Tank3/6(LL2)
  Tank3/1(LL3) -> LL3/1, Tank2/4(LL3)
  EB2/1 -> Tank2/3(EB2)
  CT2/1 -> Tank2/1(CT2)
  E3/1 -> Tank3/3(E3)
  T2/1 -> Tank2/2(T2)
  CT3/1 -> Tank3/1(CT3)
  F3/1 -> Tank3/2(F3)
  EB3/1 -> Tank3/5(EB3)
  T3/1 -> Tank3/4(T3)

== system c00016M_harness/M152 ==
  note: VALUES
      | ---------------------------------
      | ControlType = 1 | 2 | 3
      | FillTank = 0 | 1
      | EmptyTank = 0 | 1
      | ManualReference between 0 and 1
      | Tempreature between 0 and 100
      | EmergencyButton = 0 | 1
      | LiquidLevel between 0 and 1 (hmax)
  note: Inputs For Tank2
  note: NAMES
      | --------------------------------------------
      | CT1 = ControlType Tank 1
      | F1 = Fill Tank 1
      | E1 = Empty Tank 1
      | MR1 = Manual Reference Tank1
      | T1 = Temperature Tank 1
      | EB1 = Emergency Button Tank 1
      | LL1 = Liquid Level 1
  note: Inputs For Tank3
  note: Inputs For Tank1
  CT2 : Inport
  T2 : Inport  Port=2
  EB2 : Inport  Port=3
  CT3 : Inport  Port=4
  F3 : Inport  Port=5
  E3 : Inport  Port=6
  T3 : Inport  Port=7
  EB3 : Inport  Port=8
  Tank2 : Subsystem
  Tank3 : Subsystem
  LL2 : Outport
  LL3 : Outport  Port=2
  wires:
  Tank2/1(LL2) -> LL2/1, Tank3/6(LL2)
  Tank3/1(LL3) -> LL3/1, Tank2/4(LL3)
  EB2/1 -> Tank2/3(EB2)
  CT2/1 -> Tank2/1(CT2)
  E3/1 -> Tank3/3(E3)
  T2/1 -> Tank2/2(T2)
  CT3/1 -> Tank3/1(CT3)
  F3/1 -> Tank3/2(F3)
  EB3/1 -> Tank3/5(EB3)
  T3/1 -> Tank3/4(T3)

== system c00016M_harness/M153 ==
  note: VALUES
      | ---------------------------------
      | ControlType = 1 | 2 | 3
      | FillTank = 0 | 1
      | EmptyTank = 0 | 1
      | ManualReference between 0 and 1
      | Tempreature between 0 and 100
      | EmergencyButton = 0 | 1
      | LiquidLevel between 0 and 1 (hmax)
  note: Inputs For Tank2
  note: NAMES
      | --------------------------------------------
      | CT1 = ControlType Tank 1
      | F1 = Fill Tank 1
      | E1 = Empty Tank 1
      | MR1 = Manual Reference Tank1
      | T1 = Temperature Tank 1
      | EB1 = Emergency Button Tank 1
      | LL1 = Liquid Level 1
  note: Inputs For Tank3
  note: Inputs For Tank1
  CT2 : Inport
  T2 : Inport  Port=2
  EB2 : Inport  Port=3
  CT3 : Inport  Port=4
  F3 : Inport  Port=5
  E3 : Inport  Port=6
  T3 : Inport  Port=7
  EB3 : Inport  Port=8
  Tank2 : Subsystem
  Tank3 : Subsystem
  LL2 : Outport
  LL3 : Outport  Port=2
  wires:
  Tank2/1(LL2) -> LL2/1, Tank3/6(LL2)
  Tank3/1(LL3) -> LL3/1, Tank2/4(LL3)
  EB2/1 -> Tank2/3(EB2)
  CT2/1 -> Tank2/1(CT2)
  E3/1 -> Tank3/3(E3)
  T2/1 -> Tank2/2(T2)
  CT3/1 -> Tank3/1(CT3)
  F3/1 -> Tank3/2(F3)
  EB3/1 -> Tank3/5(EB3)
  T3/1 -> Tank3/4(T3)

== system c00016M_harness/M154 ==
  note: VALUES
      | ---------------------------------
      | ControlType = 1 | 2 | 3
      | FillTank = 0 | 1
      | EmptyTank = 0 | 1
      | ManualReference between 0 and 1
      | Tempreature between 0 and 100
      | EmergencyButton = 0 | 1
      | LiquidLevel between 0 and 1 (hmax)
  note: Inputs For Tank2
  note: NAMES
      | --------------------------------------------
      | CT1 = ControlType Tank 1
      | F1 = Fill Tank 1
      | E1 = Empty Tank 1
      | MR1 = Manual Reference Tank1
      | T1 = Temperature Tank 1
      | EB1 = Emergency Button Tank 1
      | LL1 = Liquid Level 1
  note: Inputs For Tank3
  note: Inputs For Tank1
  CT2 : Inport
  T2 : Inport  Port=2
  EB2 : Inport  Port=3
  CT3 : Inport  Port=4
  F3 : Inport  Port=5
  E3 : Inport  Port=6
  T3 : Inport  Port=7
  EB3 : Inport  Port=8
  Tank2 : Subsystem
  Tank3 : Subsystem
  LL2 : Outport
  LL3 : Outport  Port=2
  wires:
  Tank2/1(LL2) -> LL2/1, Tank3/6(LL2)
  Tank3/1(LL3) -> LL3/1, Tank2/4(LL3)
  EB2/1 -> Tank2/3(EB2)
  CT2/1 -> Tank2/1(CT2)
  E3/1 -> Tank3/3(E3)
  T2/1 -> Tank2/2(T2)
  CT3/1 -> Tank3/1(CT3)
  F3/1 -> Tank3/2(F3)
  EB3/1 -> Tank3/5(EB3)
  T3/1 -> Tank3/4(T3)

== system c00016M_harness/M155 ==
  note: VALUES
      | ---------------------------------
      | ControlType = 1 | 2 | 3
      | FillTank = 0 | 1
      | EmptyTank = 0 | 1
      | ManualReference between 0 and 1
      | Tempreature between 0 and 100
      | EmergencyButton = 0 | 1
      | LiquidLevel between 0 and 1 (hmax)
  note: Inputs For Tank2
  note: NAMES
      | --------------------------------------------
      | CT1 = ControlType Tank 1
      | F1 = Fill Tank 1
      | E1 = Empty Tank 1
      | MR1 = Manual Reference Tank1
      | T1 = Temperature Tank 1
      | EB1 = Emergency Button Tank 1
      | LL1 = Liquid Level 1
  note: Inputs For Tank3
  note: Inputs For Tank1
  CT2 : Inport
  T2 : Inport  Port=2
  EB2 : Inport  Port=3
  CT3 : Inport  Port=4
  F3 : Inport  Port=5
  E3 : Inport  Port=6
  T3 : Inport  Port=7
  EB3 : Inport  Port=8
  Tank2 : Subsystem
  Tank3 : Subsystem
  LL2 : Outport
  LL3 : Outport  Port=2
  wires:
  Tank2/1(LL2) -> LL2/1, Tank3/6(LL2)
  Tank3/1(LL3) -> LL3/1, Tank2/4(LL3)
  EB2/1 -> Tank2/3(EB2)
  CT2/1 -> Tank2/1(CT2)
  E3/1 -> Tank3/3(E3)
  T2/1 -> Tank2/2(T2)
  CT3/1 -> Tank3/1(CT3)
  F3/1 -> Tank3/2(F3)
  EB3/1 -> Tank3/5(EB3)
  T3/1 -> Tank3/4(T3)

== system c00016M_harness/M156 ==
  note: VALUES
      | ---------------------------------
      | ControlType = 1 | 2 | 3
      | FillTank = 0 | 1
      | EmptyTank = 0 | 1
      | ManualReference between 0 and 1
      | Tempreature between 0 and 100
      | EmergencyButton = 0 | 1
      | LiquidLevel between 0 and 1 (hmax)
  note: Inputs For Tank2
  note: NAMES
      | --------------------------------------------
      | CT1 = ControlType Tank 1
      | F1 = Fill Tank 1
      | E1 = Empty Tank 1
      | MR1 = Manual Reference Tank1
      | T1 = Temperature Tank 1
      | EB1 = Emergency Button Tank 1
      | LL1 = Liquid Level 1
  note: Inputs For Tank3
  note: Inputs For Tank1
  CT2 : Inport
  T2 : Inport  Port=2
  EB2 : Inport  Port=3
  CT3 : Inport  Port=4
  F3 : Inport  Port=5
  E3 : Inport  Port=6
  T3 : Inport  Port=7
  EB3 : Inport  Port=8
  Tank2 : Subsystem
  Tank3 : Subsystem
  LL2 : Outport
  LL3 : Outport  Port=2
  wires:
  Tank2/1(LL2) -> LL2/1, Tank3/6(LL2)
  Tank3/1(LL3) -> LL3/1, Tank2/4(LL3)
  EB2/1 -> Tank2/3(EB2)
  CT2/1 -> Tank2/1(CT2)
  E3/1 -> Tank3/3(E3)
  T2/1 -> Tank2/2(T2)
  CT3/1 -> Tank3/1(CT3)
  F3/1 -> Tank3/2(F3)
  EB3/1 -> Tank3/5(EB3)
  T3/1 -> Tank3/4(T3)

== system c00016M_harness/M157 ==
  note: VALUES
      | ---------------------------------
      | ControlType = 1 | 2 | 3
      | FillTank = 0 | 1
      | EmptyTank = 0 | 1
      | ManualReference between 0 and 1
      | Tempreature between 0 and 100
      | EmergencyButton = 0 | 1
      | LiquidLevel between 0 and 1 (hmax)
  note: Inputs For Tank2
  note: NAMES
      | --------------------------------------------
      | CT1 = ControlType Tank 1
      | F1 = Fill Tank 1
      | E1 = Empty Tank 1
      | MR1 = Manual Reference Tank1
      | T1 = Temperature Tank 1
      | EB1 = Emergency Button Tank 1
      | LL1 = Liquid Level 1
  note: Inputs For Tank3
  note: Inputs For Tank1
  CT2 : Inport
  T2 : Inport  Port=2
  EB2 : Inport  Port=3
  CT3 : Inport  Port=4
  F3 : Inport  Port=5
  E3 : Inport  Port=6
  T3 : Inport  Port=7
  EB3 : Inport  Port=8
  Tank2 : Subsystem
  Tank3 : Subsystem
  LL2 : Outport
  LL3 : Outport  Port=2
  wires:
  Tank2/1(LL2) -> LL2/1, Tank3/6(LL2)
  Tank3/1(LL3) -> LL3/1, Tank2/4(LL3)
  EB2/1 -> Tank2/3(EB2)
  CT2/1 -> Tank2/1(CT2)
  E3/1 -> Tank3/3(E3)
  T2/1 -> Tank2/2(T2)
  CT3/1 -> Tank3/1(CT3)
  F3/1 -> Tank3/2(F3)
  EB3/1 -> Tank3/5(EB3)
  T3/1 -> Tank3/4(T3)

== system c00016M_harness/M158 ==
  note: VALUES
      | ---------------------------------
      | ControlType = 1 | 2 | 3
      | FillTank = 0 | 1
      | EmptyTank = 0 | 1
      | ManualReference between 0 and 1
      | Tempreature between 0 and 100
      | EmergencyButton = 0 | 1
      | LiquidLevel between 0 and 1 (hmax)
  note: Inputs For Tank2
  note: NAMES
      | --------------------------------------------
      | CT1 = ControlType Tank 1
      | F1 = Fill Tank 1
      | E1 = Empty Tank 1
      | MR1 = Manual Reference Tank1
      | T1 = Temperature Tank 1
      | EB1 = Emergency Button Tank 1
      | LL1 = Liquid Level 1
  note: Inputs For Tank3
  note: Inputs For Tank1
  CT2 : Inport
  T2 : Inport  Port=2
  EB2 : Inport  Port=3
  CT3 : Inport  Port=4
  F3 : Inport  Port=5
  E3 : Inport  Port=6
  T3 : Inport  Port=7
  EB3 : Inport  Port=8
  Tank2 : Subsystem
  Tank3 : Subsystem
  LL2 : Outport
  LL3 : Outport  Port=2
  wires:
  Tank2/1(LL2) -> LL2/1, Tank3/6(LL2)
  Tank3/1(LL3) -> LL3/1, Tank2/4(LL3)
  EB2/1 -> Tank2/3(EB2)
  CT2/1 -> Tank2/1(CT2)
  E3/1 -> Tank3/3(E3)
  T2/1 -> Tank2/2(T2)
  CT3/1 -> Tank3/1(CT3)
  F3/1 -> Tank3/2(F3)
  EB3/1 -> Tank3/5(EB3)
  T3/1 -> Tank3/4(T3)
